simulink model "buck_interval_flatten_actual"  (R2014a)
settings: Solver=ode4  StartTime=0.0  StopTime=Inf  FixedStep=0.00002  RelTol=1e-3
PostLoadFcn:
  | , if any(exist('dsrtsu_mdlpostloadfcn', 'file') == [2, 3, 6]), try dsrtsu_mdlpostloadfcn('Execute', bdroot); catch fprintf('Error in PostLoadFcn (dsrtsu_mdlpostloadfcn) for model "%s":\n %s\n', bdroot, lasterr); end, end,
InitFcn:
  | %Tol = 0.02;
libraries: rtilib1103 x2
PreSaveFcn:
  | , if any(exist('dsmpb_private', 'file') == [2, 3, 6]), try, dsmpb_private('dsmpb_mdlclblib', 'PreSave', bdroot); catch, disp(lasterr); end, end,
CloseFcn:
  | , if any(exist('dsmpb_private', 'file') == [2, 3, 6]), try, dsmpb_private('dsmpb_mdlclblib', 'Close', bdroot); catch, disp(lasterr); end, end,
settings Model: DSRTSU_INTERNAL_RTI_VER=440  DSRTSU_INTERNAL_RTI_TYPE=rti1103  DSRTSU_INTERNAL_RTIFPGA=30  DSMPB_DATASERVER_ModelPortLibVersion1=7  DSMPB_DATASERVER_DataServerVersion1=6  DSMPB_DATASERVER_DataServerStreamVersion1=3  BufferReuse=off  Creator=Omar A Beg  LastModifiedBy=OmarAli
settings DataIOCC: SignalLoggingSaveFormat=ModelDataLogs
settings OptimizationCC: BlockReduction=off  OptimizeBlockIOStorage=off  BufferReuse=off  GlobalBufferReuse=off  ExpressionFolding=off  ExpressionDepthLimit=2147483647  LocalBlockOutputs=off
settings DebuggingCC: UnderspecifiedInitializationDetection=Classic  FcnCallInpInsideContextMsg=EnableAllAsWarning  StateNameClashWarn=warning
settings HardwareCC: ProdIntDivRoundTo=Zero  ProdEndianess=BigEndian  ProdHWDeviceType=Generic->Custom  TargetIntDivRoundTo=Zero  TargetEndianess=BigEndian  TargetHWDeviceType=Generic->Custom
settings RTWCC: SystemTargetFile=rti1103.tlc  MakeCommand=make_rti  TemplateMakefile=rti1103.tmf  Description=dSPACE DS1103 Hardware Platform  ProcessScript=rti1103_make_rtw_hook
settings STFCustomTargetCC: ParMdlRefBuildCompliant=on  ConcurrentExecutionCompliant=off  SystemTargetFile=rti1103.tlc
settings GRTTargetCC: CompOptLevelCompliant=off  ConcurrentExecutionCompliant=off  CombineOutputUpdateFcns=off  MatFileLogging=off  CPPClassGenCompliant=off  GRTInterface=on  ExtModeMexFile=noextcomm

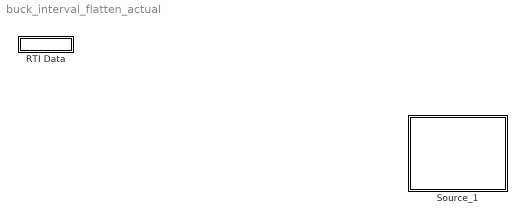
== system buck_interval_flatten_actual ==
  RTI Data : Subsystem  Tag=struct('RTIDataServer',struct('RTIDataServerVs','2','RTIModelDescription','struct(''main'',''buck_interval_flatten_actual'',''sub'','''',''isMp'',0)'))  LoadFcn="if exist('rtidc'), try,  rtidc('DataHostBlockClbLoad', gcbh); catch, disp(['Warning: ''LoadFcn'' for RTI Data block failed: ' lasterr]); end, end,"  mask(RTI_DATA_HOST){}
      mask help:
      | RTI Data Block.
      | This block is used by RTI to store internal model-dependent data.
      | Please keep this block on the root level of the model. Deleting this block will result in data loss.
      |
      | NEVER DELETE OR COPY THIS BLOCK!
      settings: CopyFcn="if exist('rtidc'), try,  rtidc('DataHostBlockClbCopy', gcbh); catch, disp(['Warning: ''CopyFcn'' for RTI Data block failed: ' lasterr]); end, end,"  DeleteFcn="if exist('rtidc'), try,  rtidc('DataHostBlockClbDelete', gcbh); catch, disp(['Warning: ''DeleteFcn'' for RTI Data block failed: ' lasterr]); end, end,"  ModelCloseFcn="if exist('rtidc'), try,  rtidc('DataHostBlockClbModelClose', gcbh); catch, disp(['Warning: ''ModelCloseFcn'' for RTI Data block failed: ' lasterr]); end, end,"  PreSaveFcn="if exist('rtidc'), try,  rtidc('DataHostBlockClbPreSave', gcbh); catch, disp(['Warning: ''PreSaveFcn'' for RTI Data block failed: ' lasterr]); end, end,"  PostSaveFcn="if exist('rtidc'), try,  rtidc('DataHostBlockClbPostSave', gcbh); catch, disp(['Warning: ''PostSaveFcn'' for RTI Data block failed: ' lasterr]); end, end,"  NameChangeFcn="if exist('rtidc'), try,  rtidc('DataHostBlockClbNameChange', gcbh); catch, disp(['Warning: ''NameChangeFcn'' for RTI Data block failed: ' lasterr]); end, end,"
      mask Help:
      | RTI Data Block.
      | This block is used by RTI to store internal model-dependent data.
      | Please keep this block on the root level of the model. Deleting this block will result in data loss.
      | 
      | NEVER DELETE OR COPY THIS BLOCK!
      mask Display:
      | text(0.5, 0.5, 'RTI Data', 'HorizontalAlignment', 'center');
      | plot([1 0]);
  Source_1 : Subsystem  mask{Kv=69.04, Ki=5.5}
      mask prompts: Kv "Voltage ADC Gain"; Ki "Current ADC Gain"

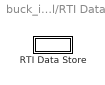
== system buck_interval_flatten_actual/RTI Data ==
  RTI Data Store : Subsystem  Tag="struct('private',struct('version',struct('dsVer',uint32(2),'dsVerCreation',uint32(2),'RTI',struct('ver','7.0','type','RTI1103')),'access',struct('type','Model','isPerm',1,'created',['03-Sep-2013 11:49:01'],'modified',['13-Jan-2016 19:35:20'],'location','')),'public',struct('main',struct('data',[]),'sub',struct('name',{{'buck_interval_flatten_actual'}},'data',{{struct('TH',struct('thTaskInfo',struct('taskType',{'TIMER','HWINT','TMRINT','SWINT','GLINT'},'tasksNumOf',{1,0,0,0,0},'srcIds',{{'TIMERA'},{},{},{},{}},'taskNames',{{['Timer Task 1']},{},{},{},{}})),'th_tc',struct('dataType','TASK','taskGroupId','','taskGroupList',{{}},'taskSchedulingPolicy','FCFS','taskType','TIMER','blkh',-1,'srcId','TIMERA','srcSgnName',['Timer A interrupt'],'srcCpuName','','taskName',['Timer Task 1  [2e-05] s'],'taskNameDisplayExt','','smplTime',2e-05,'smplTimeOffs',0,'hasFixedPriority',0,'priority',1,'hasFixedOvc',0,'ovcType',1,'ovcMax',1),'tc_th',struct('dataType','TASK','taskGroupId','','taskGroupList',{{}},'taskSchedulingPolicy','FCFS','taskType','TIMER','blkh',-1,'srcId','TIMERA','srcSgnName',['Timer A interrupt'],'srcCpuName','','taskName',['Timer Task 1  [2e-05] s'],'taskNameDisplayExt','','smplTime',2e-05,'smplTimeOffs',0,'hasFixedPriority',0,'priority',1,'hasFixedOvc',0,'ovcType',1,'ovcMax',1))}})))"  mask(RTI_DATA_STORE){}
      mask help:
      | RTI Data Store Block. This block is used by RTI to store internal model dependent data. Deleting this block will result in data loss.
      |
      | NEVER DELETE, COPY, OR MODIFY THIS BLOCK!
      mask Help:
      | RTI Data Store Block. This block is used by RTI to store internal model dependent data. Deleting this block will result in data loss.
      | 
      | NEVER DELETE, COPY, OR MODIFY THIS BLOCK!
      mask Display: text(0.5, 0.5, ' ', 'HorizontalAlignment', 'center');

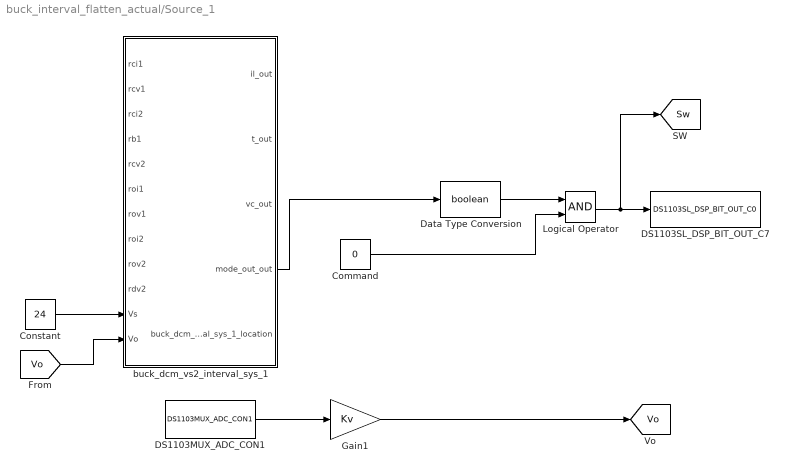
== system buck_interval_flatten_actual/Source_1 ==
  Command : Constant  Value=0  OutDataTypeStr=boolean
  Constant : Constant  Value=24
  DS1103MUX_ADC_CON1 : rtilib1103/DS1103 MASTER PPC/DS1103MUX_ADC_CON1  ConverterNo=1  ChannelNos=1  TimerAPreTrigger=0  Reserved2=[]  Reserved3=[]  Reserved4=[]  DialogFcn=gui1103mux_adc  UnitName={ 'DS1103MUX_ADC_CON' }  UnitValues={ 1 }  DSProperties=struct('RTI',struct('Version',uint32(1),'BlockType',struct('isSLSource',uint8(1),'isSLSink',uint8(0),'isHWSource',uint8(1),'isHWSink',uint8(0),'isSetup',uint8(0),'isInline',uint8(1),'isNonInline',uint8(0),'isInterrupt',uint8(0),'isChannelwise',uint8(0)),'IOBoardType','DS1103MASTER','UnitType','ADC','Identifier','ADCMUX','DialogType','ML','BlockSet','NONE','SlaveProcessor','NONE'))
  DS1103SL_DSP_BIT_OUT_C7 : rtilib1103/DS1103 SLAVE DSP/DS1103SL_DSP_BIT_OUT_C0  ChannelNo=7  InitValue=0  TermMode=0  TermValue=0  Reserved1=[]  Reserved2=[]  Reserved3=[]  Reserved=[]  DialogFcn=gui1103sl_dsp_bit_out  UnitName={ 'DS1103SL_DSP_BIT_OUT_C'}  UnitValues={ 7 }  DSProperties=struct('RTI',struct('Version',uint32(1),'BlockType',struct('isSLSource',uint8(0),'isSLSink',uint8(1),'isHWSource',uint8(0),'isHWSink',uint8(1),'isSetup',uint8(0),'isInline',uint8(1),'isNonInline',uint8(0),'isInterrupt',uint8(0),'isChannelwise',uint8(1)),'IOBoardType','DS1103SLAVE','UnitType','BIT','Identifier','BITOUTCH','DialogType','ML','BlockSet','NONE','SlaveProcessor','F240'))
  Data Type Conversion : DataTypeConversion  OutDataTypeStr=boolean
  Gain1 : Gain  Gain=Kv
  Logical Operator : Logic  AllPortsSameDT=off  OutDataTypeStr=boolean
  buck_dcm_vs2_interval_sys_1 : Stateflow chart  TreatAsAtomicUnit=on
  tag scope: Sw=global, Vo=global
  wires:
  DS1103MUX_ADC_CON1/1 -> Gain1/1
  Gain1/1 -> [Vo]
  [Vo] -> buck_dcm_vs2_interval_sys_1/12(Vo)
  Data Type Conversion/1 -> Logical Operator/1
  Logical Operator/1 -> [Sw], DS1103SL_DSP_BIT_OUT_C7/1
  Command/1 -> Logical Operator/2
  buck_dcm_vs2_interval_sys_1/4(mode_out_out) -> Data Type Conversion/1
  Constant/1 -> buck_dcm_vs2_interval_sys_1/11(Vs)

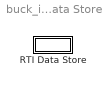
== system buck_interval_flatten_actual/RTI Data/RTI Data Store ==
  RTI Data Store : Subsystem  mask(RTI_DATA_STORE){}
      mask help:
      | RTI Data Store Block. This block is used by RTI to store internal model dependent data. Deleting this block will result in data loss.
      |
      | NEVER DELETE, COPY, OR MODIFY THIS BLOCK!
      mask Help:
      | RTI Data Store Block. This block is used by RTI to store internal model dependent data. Deleting this block will result in data loss.
      | 
      | NEVER DELETE, COPY, OR MODIFY THIS BLOCK!
      mask Display: text(0.5, 0.5, ' ', 'HorizontalAlignment', 'center');

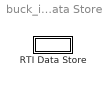
== system buck_interval_flatten_actual/RTI Data/RTI Data Store/RTI Data Store ==
  RTI Data Store : Subsystem  mask(RTI_DATA_STORE){}
      mask help:
      | RTI Data Store Block. This block is used by RTI to store internal model dependent data. Deleting this block will result in data loss.
      |
      | NEVER DELETE, COPY, OR MODIFY THIS BLOCK!
      mask Help:
      | RTI Data Store Block. This block is used by RTI to store internal model dependent data. Deleting this block will result in data loss.
      | 
      | NEVER DELETE, COPY, OR MODIFY THIS BLOCK!
      mask Display: text(0.5, 0.5, ' ', 'HorizontalAlignment', 'center');

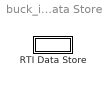
== system buck_interval_flatten_actual/RTI Data/RTI Data Store/RTI Data Store/RTI Data Store ==
  RTI Data Store : Subsystem  mask(RTI_DATA_STORE){}
      mask help:
      | RTI Data Store Block. This block is used by RTI to store internal model dependent data. Deleting this block will result in data loss.
      |
      | NEVER DELETE, COPY, OR MODIFY THIS BLOCK!
      mask Help:
      | RTI Data Store Block. This block is used by RTI to store internal model dependent data. Deleting this block will result in data loss.
      | 
      | NEVER DELETE, COPY, OR MODIFY THIS BLOCK!
      mask Display: text(0.5, 0.5, ' ', 'HorizontalAlignment', 'center');

== system buck_interval_flatten_actual/RTI Data/RTI Data Store/RTI Data Store/RTI Data Store/RTI Data Store ==

== stateflow chart buck_interval_flatten_actual/Source_1/buck_dcm_vs2_interval_sys_1 ==
  settings: updateMethod=CONTINUOUS
  state charging_charging_controller
    du:
    il_dot = buckboost_template_1_a00c * il + rci1 + buckboost_template_1_a01c * vc + rcv1 + buckboost_template_1_b0c * Vs + rb1;
    vc_dot = buckboost_template_1_a10c * il + rci2 + buckboost_template_1_a11c * vc + rcv2 + buckboost_template_1_b1c * Vs;
    t_dot = 1;
    mode_out_dot = 0;
    il_out=il;
    t_out=t;
    vc_out=vc;
    mode_out_out=mode_out;
    buck_dcm_vs2_interval_sys_1_location =1;
  state discharging_discharging_controller
    du:
    il_dot = buckboost_template_1_a00o * il + roi1 + buckboost_template_1_a01o * vc + rov1 + buckboost_template_1_b0o * Vs;
    vc_dot = buckboost_template_1_a10o * il + roi2 + buckboost_template_1_a11o * vc + rov2 + buckboost_template_1_b1o * Vs;
    t_dot = 1;
    mode_out_dot = 0;
    il_out=il;
    t_out=t;
    vc_out=vc;
    mode_out_out=mode_out;
    buck_dcm_vs2_interval_sys_1_location =2;
  state dcm_discharging_controller
    du:
    il_dot = 0;
    vc_dot = buckboost_template_1_a11o * vc + rdv2 + buckboost_template_1_b1o * Vs;
    t_dot = 1;
    mode_out_dot = 0;
    il_out=il;
    t_out=t;
    vc_out=vc;
    mode_out_out=mode_out;
    buck_dcm_vs2_interval_sys_1_location =3;
  charging_charging_controller -> discharging_discharging_controller : [Vo >= VcH]
      | {mode_out = 0;}
  discharging_discharging_controller -> dcm_discharging_controller [order 2] : [il <= 0 && Vo > VcL]
  (default) -> charging_charging_controller : {il = 0;
      | vc = 0;
      | t = 0;
      | mode_out = 1;}
  discharging_discharging_controller -> charging_charging_controller [order 1] : [Vo <= VcL]
      | {mode_out = 1;}
  dcm_discharging_controller -> charging_charging_controller : [Vo <= VcL]
      | {mode_out = 1;}
  data: il_out output; il local; t_out output; t local; vc_out output; vc local; mode_out_out output; mode_out local; rci1 input; rcv1 input; rci2 input; rb1 input; rcv2 input; roi1 input; rov1 input; roi2 input; rov2 input; rdv2 input; buck_dcm_vs2_interval_sys_1_location output; VcH constant double =12.1; buckboost_template_1_a11o constant double =-45.4545; tmax constant double =0.0375; buckboost_template_1_a01o constant double =-377.3585; VcL constant double =11.9; buckboost_template_1_a10o constant double =454.5455; Vs input double =24; buckboost_template_1_a00o constant double =-196.2264; buckboost_template_1_b1o constant double =0; buckboost_template_1_b0o constant double =0; buckboost_template_1_a11c constant double =-45.4545; buckboost_template_1_b0c constant double =377.3585; buckboost_template_1_a10c constant double =454.5455; buckboost_template_1_b1c constant double =0; buckboost_template_1_bounds constant double =1000; buckboost_template_1_a01c constant double =-377.3585; buckboost_template_1_a00c constant double =-271.6981; Vo input
  data il settings: updateMethod=SF_CONTINUOUS_TIME_DATA
  data t settings: updateMethod=SF_CONTINUOUS_TIME_DATA
  data vc settings: updateMethod=SF_CONTINUOUS_TIME_DATA
  data mode_out settings: updateMethod=SF_CONTINUOUS_TIME_DATA
  data rci1 settings: updateMethod=SF_CONTINUOUS_TIME_DATA
  data rcv1 settings: updateMethod=SF_CONTINUOUS_TIME_DATA
  data rci2 settings: updateMethod=SF_CONTINUOUS_TIME_DATA
  data rb1 settings: updateMethod=SF_CONTINUOUS_TIME_DATA
  data rcv2 settings: updateMethod=SF_CONTINUOUS_TIME_DATA
  data roi1 settings: updateMethod=SF_CONTINUOUS_TIME_DATA
  data rov1 settings: updateMethod=SF_CONTINUOUS_TIME_DATA
  data roi2 settings: updateMethod=SF_CONTINUOUS_TIME_DATA
  data rov2 settings: updateMethod=SF_CONTINUOUS_TIME_DATA
  data rdv2 settings: updateMethod=SF_CONTINUOUS_TIME_DATA
